simulink model "sampleModel1648"  (R2023a)
settings: Solver=VariableStepAuto  StartTime=0.0  StopTime=10.0  RelTol=1e-3
libraries: hdlsllib x2, simulink x1
settings Model: Creator=user1  LastModifiedBy=user1

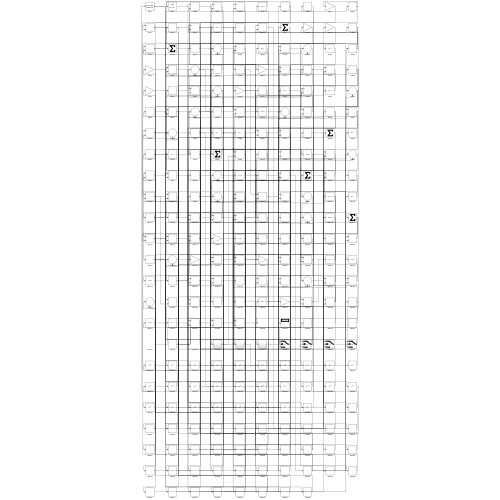
[thumbnail: Simulink's stored preview of the top-level diagram]
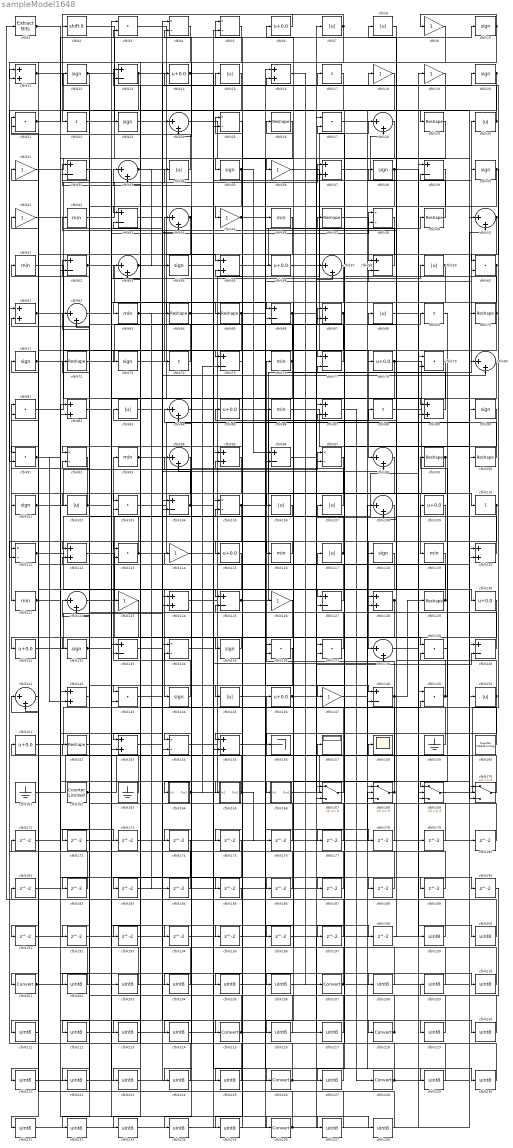
== system sampleModel1648 ==
  cfblk1 : simulink/Logic and Bit Operations/Extract Bits  bitsToExtract=Upper half  numBits=8  bitIdxRange=[0 7]  outScalingMode=Preserve fixed-point scaling
      settings: LibrarySourceBlock=|
      | hdlsllib/Logic and Bit
      | Operations/Extract Bits
  cfblk{10,12,20,23,35,38,40,54,71,73,90,101,118,132,135,144} (16 alike) : Signum
  cfblk{26,29,47,49,64..65,70,72,99..100,129,152} (12 alike) : Reshape
  cfblk{7..8,15,30,34,59,68,83,102,106..107,117,145,150} (14 alike) : Abs  SaturateOnIntegerOverflow=off
  cfblk{3,21,27,60,79,81,91,103,113,136..137,139,143,149} (14 alike) : DotProduct  OutDataTypeStr=Inherit: Inherit via internal rule
  cfblk{13,32,39,43,52,58,66,75,77,96,104,125,127,133,140,148} (16 alike) : Sum  Inputs=+-
  cfblk{4..5,25,48,92,97,105,111,134,154} (10 alike) : Product  Inputs=*/  RndMeth=Zero  SaturateOnIntegerOverflow=on
  cfblk{24,28,33,44,50,53,57,62,80,84,94,98,108,122,138,141} (16 alike) : Sum  Inputs=|++
  cfblk{6,14,56,78,85,109,115,130..131,146,151} (11 alike) : Bias  Bias=0.0  SaturateOnIntegerOverflow=off
  cfblk{11,16,37,55,61,67,82,87,89,95,112,120,124,128,142,153,155} (17 alike) : Sum
  cfblk{17,22,69,74,88,110} (6 alike) : Sum  Inputs=+
  cfblk{9,18..19,31,36,41,45,114,123,126,147} (11 alike) : Gain
  cfblk{42,46,51,63,76,86,93,116,119,121} (10 alike) : MinMax
  cfblk156 : Terminator
  cfblk157 : Display
  cfblk158 : Scope
  cfblk159 : Ground
  cfblk160 : hdlsllib/Sources/Counter Free-Running  NumBits=16  tsamp=-1
  cfblk161 : Ground
  cfblk162 : hdlsllib/Sources/Counter Limited  uplimit=7  tsamp=-1
  cfblk163 : Ground
  cfblk164 : Subsystem
      settings: LibrarySourceBlock=|
      | hdlsllib/Ports &
      | Subsystems/Subsystem
  cfblk165 : Subsystem
      settings: LibrarySourceBlock=|
      | hdlsllib/Ports &
      | Subsystems/Subsystem
  cfblk166 : Subsystem
      settings: LibrarySourceBlock=|
      | hdlsllib/Ports &
      | Subsystems/Subsystem
  cfblk{167..170} (4 alike) : Switch  SaturateOnIntegerOverflow=off  InputSameDT=off
  cfblk{171..198} (28 alike) : Delay  SampleTime=1
  cfblk{199..200,202..206,208..214,216..217,219..225,227,229..235,237..238} (33 alike) : DataTypeConversion  OutDataTypeStr=uint8  SaturateOnIntegerOverflow=off  RndMeth=Floor
  cfblk2 : ArithShift  BitShiftNumber=8
  cfblk{201,207,215,218,226,228,236} (7 alike) : DataTypeConversion  SaturateOnIntegerOverflow=off  RndMeth=Floor
  wires:
  cfblk78/1 -> cfblk110/1, cfblk153/1
  cfblk31/1 -> cfblk35/1
  cfblk33/1 -> cfblk55/1, cfblk54/1, cfblk13/2
  cfblk101/1 -> cfblk97/1, cfblk154/2
  cfblk22/1 -> cfblk10/1
  cfblk26/1 -> cfblk92/1
  cfblk92/1 -> cfblk121/1
  cfblk3/1 -> cfblk77/1
  cfblk59/1 -> cfblk63/1, cfblk177/1
  cfblk148/1 -> cfblk76/1, cfblk129/1, cfblk206/1
  cfblk125/1 -> cfblk30/1, cfblk148/1
  cfblk166/1(Out1) -> cfblk158/1
  cfblk144/1 -> cfblk93/1
  cfblk108/1 -> cfblk138/1
  cfblk98/1 -> cfblk131/1
  cfblk6/1 -> cfblk22/1
  cfblk7/1 -> cfblk2/1, cfblk11/2, cfblk104/2
  cfblk11/1 -> cfblk50/1, cfblk220/1
  cfblk100/1 -> cfblk84/1
  cfblk169/1 -> cfblk15/1
  cfblk29/1 -> cfblk147/1
  cfblk42/1 -> cfblk34/1
  cfblk36/1 -> cfblk98/1
  cfblk2/1 -> cfblk126/1
  cfblk114/1 -> cfblk226/1
  cfblk54/1 -> cfblk40/1
  cfblk105/1 -> cfblk88/1, cfblk164/1(In1), cfblk60/2, cfblk174/1
  cfblk70/1 -> cfblk143/1, cfblk47/1
  cfblk133/1 -> cfblk215/1
  cfblk164/1(Out1) -> cfblk28/1, cfblk75/2
  cfblk44/1 -> cfblk84/2, cfblk202/1
  cfblk14/1 -> cfblk29/1, cfblk116/1
  cfblk8/1 -> cfblk128/1
  cfblk150/1 -> cfblk107/1, cfblk216/1
  cfblk97/1 -> cfblk106/1
  cfblk106/1 -> cfblk105/2
  cfblk81/1 -> cfblk37/1
  cfblk115/1 -> cfblk144/1
  cfblk85/1 -> cfblk119/1
  cfblk35/1 -> cfblk45/1, cfblk96/1, cfblk124/2
  cfblk83/1 -> cfblk98/2
  cfblk56/1 -> cfblk28/2
  cfblk116/1 -> cfblk115/1
  cfblk53/1 -> cfblk89/1, cfblk139/1
  cfblk124/1 -> cfblk70/1
  cfblk65/1 -> cfblk111/1, cfblk48/1
  cfblk73/1 -> cfblk44/1
  cfblk64/1 -> cfblk138/2, cfblk189/1
  cfblk13/1 -> cfblk167/2, cfblk170/2, cfblk222/1
  cfblk16/1 -> cfblk207/1
  cfblk165/1(Out1) -> cfblk112/2, cfblk176/1
  cfblk1/1 -> cfblk37/2, cfblk168/3
  cfblk140/1 -> cfblk12/1
  cfblk48/1 -> cfblk103/1
  cfblk168/1 -> cfblk33/2, cfblk96/2
  cfblk72/1 -> cfblk67/1
  cfblk50/1 -> cfblk101/1, cfblk52/2, cfblk170/3
  cfblk5/1 -> cfblk43/1
  cfblk96/1 -> cfblk69/1
  cfblk63/1 -> cfblk65/1, cfblk184/1
  cfblk154/1 -> cfblk117/1
  cfblk86/1 -> cfblk120/1
  cfblk55/1 -> cfblk49/1
  cfblk170/1 -> cfblk146/1
  cfblk47/1 -> cfblk58/1
  cfblk113/1 -> cfblk50/2, cfblk52/1
  cfblk167/1 -> cfblk25/1
  cfblk99/1 -> cfblk191/1, cfblk224/1
  cfblk37/1 -> cfblk168/1
  cfblk139/1 -> cfblk99/1
  cfblk112/1 -> cfblk135/1
  cfblk121/1 -> cfblk165/1(In1), cfblk185/1, cfblk186/1
  cfblk24/1 -> cfblk36/1
  cfblk162/1 -> cfblk74/1, cfblk157/1, cfblk108/1
  cfblk43/1 -> cfblk80/2
  cfblk19/1 -> cfblk73/1
  cfblk62/1 -> cfblk236/1
  cfblk52/1 -> cfblk66/1, cfblk192/1
  cfblk159/1 -> cfblk97/2
  cfblk141/1 -> cfblk201/1
  cfblk10/1 -> cfblk9/1, cfblk24/2
  cfblk91/1 -> cfblk142/1, cfblk142/2
  cfblk122/1 -> cfblk19/1
  cfblk149/1 -> cfblk42/1, cfblk139/2, cfblk109/1
  cfblk107/1 -> cfblk32/1
  cfblk103/1 -> cfblk57/1
  cfblk102/1 -> cfblk81/1, cfblk198/1
  cfblk51/1 -> cfblk149/1
  cfblk131/1 -> cfblk44/2
  cfblk163/1 -> cfblk81/2
  cfblk9/1 -> cfblk91/1
  cfblk38/1 -> cfblk102/1, cfblk200/1
  cfblk61/1 -> cfblk17/1, cfblk128/2
  cfblk161/1 -> cfblk120/2
  cfblk134/1 -> cfblk218/1
  cfblk129/1 -> cfblk31/1, cfblk8/1
  cfblk20/1 -> cfblk148/2, cfblk193/1
  cfblk137/1 -> cfblk61/2
  cfblk57/1 -> cfblk156/1
  cfblk67/1 -> cfblk113/1, cfblk214/1
  cfblk160/1 -> cfblk5/1
  cfblk89/1 -> cfblk6/1
  cfblk49/1 -> cfblk39/2
  cfblk18/1 -> cfblk127/1
  cfblk132/1 -> cfblk59/1, cfblk48/2
  cfblk60/1 -> cfblk143/2, cfblk225/1
  cfblk127/1 -> cfblk86/1
  cfblk74/1 -> cfblk51/1
  cfblk128/1 -> cfblk108/2, cfblk196/1
  cfblk30/1 -> cfblk18/1, cfblk13/1
  cfblk45/1 -> cfblk56/1, cfblk130/1
  cfblk17/1 -> cfblk82/2
  cfblk27/1 -> cfblk118/1
  cfblk66/1 -> cfblk75/1, cfblk58/2
  cfblk120/1 -> cfblk85/1
  cfblk77/1 -> cfblk14/1
  cfblk40/1 -> cfblk78/1, cfblk94/2, cfblk60/1
  cfblk23/1 -> cfblk90/1
  cfblk15/1 -> cfblk91/2
  cfblk151/1 -> cfblk149/2
  cfblk146/1 -> cfblk20/1, cfblk140/2
  cfblk93/1 -> cfblk57/2, cfblk127/2
  cfblk76/1 -> cfblk155/1, cfblk32/2, cfblk153/2
  cfblk117/1 -> cfblk53/1, cfblk103/2
  cfblk88/1 -> cfblk140/1
  cfblk130/1 -> cfblk154/1
  cfblk87/1 -> cfblk228/1
  cfblk135/1 -> cfblk132/1
  cfblk80/1 -> cfblk125/1
  cfblk58/1 -> cfblk26/1
  cfblk34/1 -> cfblk21/1
  cfblk110/1 -> cfblk111/2, cfblk205/1
  cfblk21/1 -> cfblk3/2, cfblk173/1
  cfblk12/1 -> cfblk66/2, cfblk112/1
  cfblk69/1 -> cfblk169/1
  cfblk126/1 -> cfblk145/1
  cfblk143/1 -> cfblk24/1
  cfblk71/1 -> cfblk155/2, cfblk237/1
  cfblk111/1 -> cfblk23/1, cfblk169/3
  cfblk41/1 -> cfblk169/2
  cfblk104/1 -> cfblk166/1(In1), cfblk94/1
  cfblk119/1 -> cfblk172/1
  cfblk172/1 -> cfblk80/1
  cfblk173/1 -> cfblk168/2
  cfblk75/1 -> cfblk175/1
  cfblk176/1 -> cfblk3/1
  cfblk177/1 -> cfblk33/1
  cfblk155/1 -> cfblk178/1
  cfblk178/1 -> cfblk92/2
  cfblk179/1 -> cfblk137/1
  cfblk180/1 -> cfblk43/2
  cfblk142/1 -> cfblk182/1
  cfblk182/1 -> cfblk61/1
  cfblk94/1 -> cfblk183/1
  cfblk183/1 -> cfblk167/1
  cfblk184/1 -> cfblk21/2
  cfblk185/1 -> cfblk1/1
  cfblk186/1 -> cfblk125/2
  cfblk28/1 -> cfblk187/1
  cfblk187/1 -> cfblk105/1
  cfblk84/1 -> cfblk188/1
  cfblk188/1 -> cfblk77/2
  cfblk189/1 -> cfblk82/1
  cfblk138/1 -> cfblk190/1
  cfblk191/1 -> cfblk167/3
  cfblk192/1 -> cfblk25/2
  cfblk193/1 -> cfblk39/1
  cfblk32/1 -> cfblk194/1
  cfblk194/1 -> cfblk67/2
  cfblk153/1 -> cfblk195/1
  cfblk109/1 -> cfblk197/1
  cfblk197/1 -> cfblk55/2
  cfblk198/1 -> cfblk38/1
  cfblk68/1 -> cfblk199/1
  cfblk199/1 -> cfblk83/1
  cfblk200/1 -> cfblk68/1
  cfblk201/1 -> cfblk181/1, cfblk180/1
  cfblk202/1 -> cfblk141/1
  cfblk152/1 -> cfblk203/1
  cfblk203/1 -> cfblk141/2
  cfblk79/1 -> cfblk204/1
  cfblk204/1 -> cfblk122/1
  cfblk205/1 -> cfblk79/1
  cfblk206/1 -> cfblk79/2
  cfblk207/1 -> cfblk122/2, cfblk89/2, cfblk151/1
  cfblk82/1 -> cfblk208/1
  cfblk208/1 -> cfblk16/1
  cfblk190/1 -> cfblk209/1
  cfblk209/1 -> cfblk16/2
  cfblk171/1 -> cfblk210/1
  cfblk210/1 -> cfblk27/2
  cfblk118/1 -> cfblk211/1
  cfblk211/1 -> cfblk171/1
  cfblk136/1 -> cfblk212/1
  cfblk212/1 -> cfblk5/2
  cfblk174/1 -> cfblk213/1
  cfblk213/1 -> cfblk136/1
  cfblk214/1 -> cfblk136/2
  cfblk215/1 -> cfblk72/1, cfblk27/1
  cfblk216/1 -> cfblk133/1
  cfblk196/1 -> cfblk217/1
  cfblk217/1 -> cfblk133/2
  cfblk218/1 -> cfblk113/2, cfblk124/1
  cfblk145/1 -> cfblk219/1
  cfblk219/1 -> cfblk134/1
  cfblk220/1 -> cfblk134/2
  cfblk123/1 -> cfblk221/1
  cfblk221/1 -> cfblk7/1
  cfblk222/1 -> cfblk123/1
  cfblk4/1 -> cfblk223/1
  cfblk223/1 -> cfblk64/1
  cfblk224/1 -> cfblk4/1
  cfblk225/1 -> cfblk4/2
  cfblk226/1 -> cfblk104/1, cfblk71/1
  cfblk90/1 -> cfblk227/1
  cfblk227/1 -> cfblk114/1
  cfblk228/1 -> cfblk100/1, cfblk170/1, cfblk53/2, cfblk11/1
  cfblk147/1 -> cfblk229/1
  cfblk229/1 -> cfblk87/1
  cfblk195/1 -> cfblk230/1
  cfblk230/1 -> cfblk87/2
  cfblk46/1 -> cfblk231/1
  cfblk231/1 -> cfblk150/1
  cfblk39/1 -> cfblk232/1
  cfblk232/1 -> cfblk46/1
  cfblk95/1 -> cfblk233/1
  cfblk233/1 -> cfblk137/2
  cfblk175/1 -> cfblk234/1
  cfblk234/1 -> cfblk95/1
  cfblk25/1 -> cfblk235/1
  cfblk235/1 -> cfblk95/2
  cfblk236/1 -> cfblk179/1, cfblk41/1, cfblk152/1
  cfblk237/1 -> cfblk62/1
  cfblk181/1 -> cfblk238/1
  cfblk238/1 -> cfblk62/2

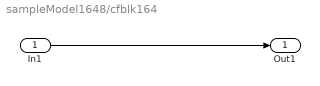
== system sampleModel1648/cfblk164 ==
  In1 : Inport
  Out1 : Outport
  wires:
  In1/1 -> Out1/1

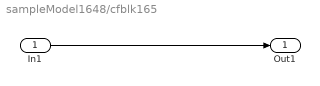
== system sampleModel1648/cfblk165 ==
  In1 : Inport
  Out1 : Outport
  wires:
  In1/1 -> Out1/1

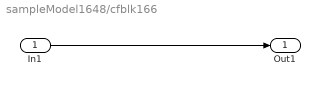
== system sampleModel1648/cfblk166 ==
  In1 : Inport
  Out1 : Outport
  wires:
  In1/1 -> Out1/1
